simulink library "INT_PTODi_TrqComp"  (R2016b)
settings: Solver=VariableStepAuto  StartTime=0.0  StopTime=10.0  RelTol=1e-3
settings Model: Creator=Administrator  LastModifiedBy=Administrator

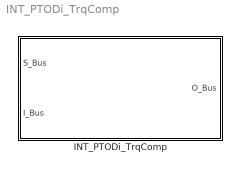
== system INT_PTODi_TrqComp ==
  INT_PTODi_TrqComp : Subsystem

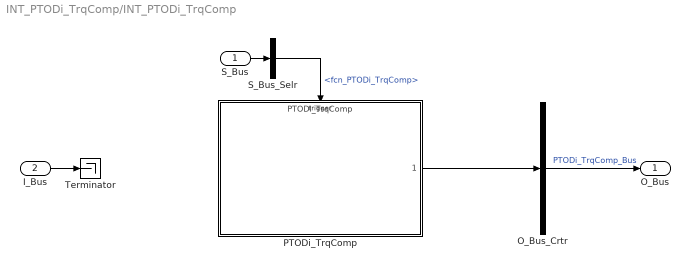
== system INT_PTODi_TrqComp/INT_PTODi_TrqComp ==
  S_Bus : Inport
  I_Bus : Inport  Port=2
  O_Bus_Crtr : BusCreator  Inputs=1
  PTODi_TrqComp : ModelReference  ModelNameDialog=PTODi_TrqComp  SimulationMode=Normal  ModelReferenceVersion=1.2  TriggerPortName=function  TriggerPortTriggerType=function-call  TriggerPortStatesWhenEnabling=held
  S_Bus_Selr : BusSelector  OutputSignals=fcn_PTODi_TrqComp
  Terminator : Terminator
  O_Bus : Outport
  wires:
  S_Bus_Selr/1 -> PTODi_TrqComp/Trigger  "<fcn_PTODi_TrqComp>"
  S_Bus/1 -> S_Bus_Selr/1
  I_Bus/1 -> Terminator/1
  O_Bus_Crtr/1 -> O_Bus/1  "PTODi_TrqComp_Bus"
  PTODi_TrqComp/1 -> O_Bus_Crtr/1
